simulink model "Pos_y_fza_P"  (R2021a)
settings: Solver=FixedStepAuto  StartTime=0.0  StopTime=Inf  FixedStep=0.01  RelTol=1e-3  EnableMultiTasking=on
libraries: arduinolib x7, cstblocks x1
settings Model: SILPILModeSetting=veronly  ExtModeTrigDuration=2  Creator=Simón  LastModifiedBy=Simón
settings OptimizationCC: EnhancedBackFolding=on  PassReuseOutputArgsAs=Individual arguments  ZeroExternalMemoryAtStartup=off  ZeroInternalMemoryAtStartup=off  MaxStackSize=64  OptimizeBlockOrder=speed  DifferentSizesBufferReuse=on  OptimizationCustomize=off  EfficientTunableParamExpr=on
settings DebuggingCC: ParameterTunabilityLossMsg=error
settings HardwareCC: ProdBitPerInt=16  ProdBitPerPointer=16  ProdBitPerSizeT=16  ProdBitPerPtrDiffT=16  ProdLargestAtomicFloat=None  ProdWordSize=8  ProdHWDeviceType=Atmel->AVR  UseEmbeddedCoderFeatures=off  UseSimulinkCoderFeatures=off
settings SFSimCC: MATLABDynamicMemAlloc=off
settings RTWCC: SystemTargetFile=ert.tlc  HardwareBoard=Arduino Uno  TemplateMakefile=ert_default_tmf  Toolchain=Arduino AVR  BuildConfiguration=Faster Runs
settings CodeAppCC: ForceParamTrailComments=on  IgnoreCustomStorageClasses=off  OperatorAnnotations=on  SimulinkDataObjDesc=on  SFDataObjDesc=on  InsertBlockDesc=on
settings ERTTargetCC: SupportContinuousTime=on  SupportNonInlinedSFcns=on  SupportVariableSizeSignals=on  ExtModeStaticAllocSize=250

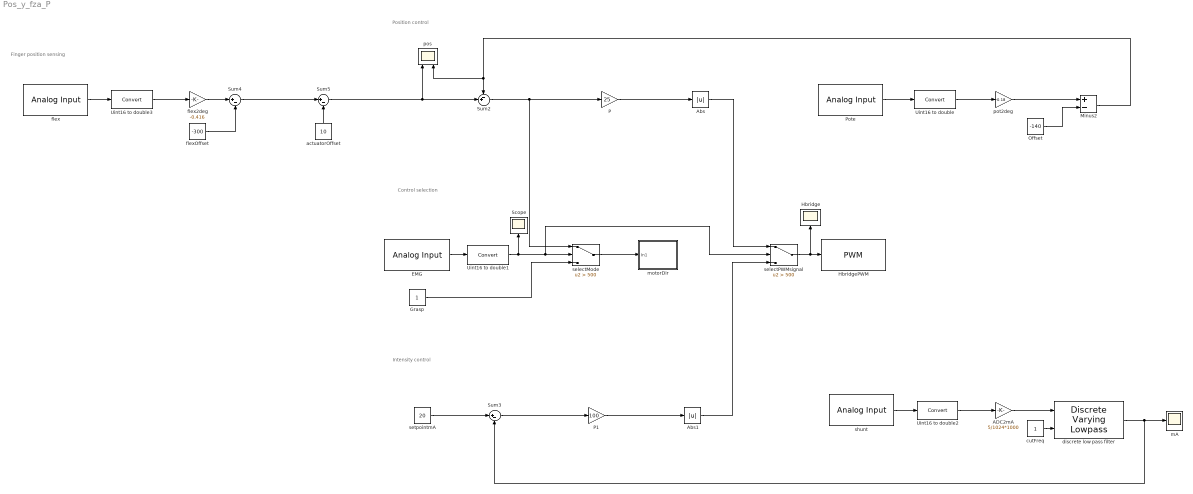
== system Pos_y_fza_P ==
  note: Finger position sensing
  note: Control selection
  note: Intensity control
  note: Position control
  ADC2mA : Gain  Gain=5/1024*1000
  Abs : Abs
  Abs1 : Abs
  EMG : arduinolib/Analog Input  pinNumber=5  ReadResultsOnly=off  ConversionTriggerSource=Software  ExternalTriggerType=uint32( 0 )  OutputDataType=uint16  EnableConversionCompleteNotify=off  EnableOuputStatus=off  SampleTime=-1  blockPlatform=arduino
  Grasp : Constant
  Hbridge : Scope
  HbridgePWM : arduinolib/PWM  pinNumber=10  frequencyType=Default  desiredFrequency=490.2  achievableFrequency=490.2
  Minus2 : Sum  Inputs=+-
  Offset : Constant  Value=-140
  P : Gain  Gain=25
  P1 : Gain  Gain=100
  Pote : arduinolib/Analog Input  pinNumber=0  ReadResultsOnly=off  ConversionTriggerSource=Software  ExternalTriggerType=uint32( 0 )  OutputDataType=uint16  EnableConversionCompleteNotify=off  EnableOuputStatus=off  SampleTime=-1  blockPlatform=arduino
  Scope : Scope
  Sum2 : Sum  Inputs=-+|
  Sum3 : Sum  Inputs=|+-
  Sum4 : Sum  Inputs=|+-
  Sum5 : Sum  Inputs=|+-
  Uint16 to double{,1..3} (4 alike) : DataTypeConversion
  actuatorOffset : Constant  Value=10
  cutFreq : Constant
  discrete low pass filter : cstblocks/Linear Parameter Varying/Discrete Varying Lowpass  N=1  w0=0  Ts=0.01
      settings: SourceProductBaseCode=CT
  flex : arduinolib/Analog Input  pinNumber=1  ReadResultsOnly=off  ConversionTriggerSource=Software  ExternalTriggerType=uint32( 0 )  OutputDataType=uint16  EnableConversionCompleteNotify=off  EnableOuputStatus=off  SampleTime=-1  blockPlatform=arduino
  flex2deg : Gain  Gain=-0.416
  flexOffset : Constant  Value=-300
  mA : Scope
  motorDir : Subsystem
  pos : Scope  NumInputPorts=2
  pot2deg : Gain  Gain=-0.18
  selectMode : Switch  Criteria=u2 > Threshold  Threshold=500
  selectPWMsignal : Switch  Criteria=u2 > Threshold  Threshold=500
  setpointmA : Constant  Value=20
  shunt : arduinolib/Analog Input  pinNumber=2  ReadResultsOnly=off  ConversionTriggerSource=Software  ExternalTriggerType=uint32( 0 )  OutputDataType=uint16  EnableConversionCompleteNotify=off  EnableOuputStatus=off  SampleTime=-1  blockPlatform=arduino
  wires:
  Pote/1 -> Uint16 to double/1
  Minus2/1 -> pos/2, Sum2/1
  Sum2/1 -> selectMode/1, P/1
  Abs/1 -> selectPWMsignal/1
  cutFreq/1 -> discrete low pass filter/2
  ADC2mA/1 -> discrete low pass filter/1
  discrete low pass filter/1 -> Sum3/2, mA/1
  shunt/1 -> Uint16 to double2/1
  Uint16 to double2/1 -> ADC2mA/1
  Uint16 to double/1 -> pot2deg/1
  pot2deg/1 -> Minus2/1
  selectMode/1 -> motorDir/1(In1)
  EMG/1 -> Uint16 to double1/1
  Uint16 to double1/1 -> Scope/1, selectPWMsignal/2, selectMode/2
  Grasp/1 -> selectMode/3
  selectPWMsignal/1 -> Hbridge/1, HbridgePWM/1
  Abs1/1 -> selectPWMsignal/3
  Sum3/1 -> P1/1
  setpointmA/1 -> Sum3/1
  flex2deg/1 -> Sum4/1
  flexOffset/1 -> Sum4/2
  flex/1 -> Uint16 to double3/1
  actuatorOffset/1 -> Sum5/2
  Offset/1 -> Minus2/2
  Uint16 to double3/1 -> flex2deg/1
  Sum4/1 -> Sum5/1
  Sum5/1 -> Sum2/2, pos/1
  P/1 -> Abs/1
  P1/1 -> Abs1/1

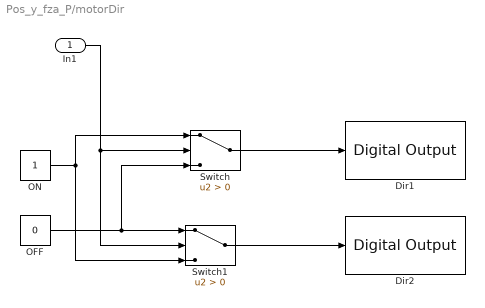
== system Pos_y_fza_P/motorDir ==
  In1 : Inport
  Dir1 : arduinolib/Digital Output  pinNumber=8  Direction=output  blockPlatform=arduino
  Dir2 : arduinolib/Digital Output  pinNumber=9  Direction=output  blockPlatform=arduino
  OFF : Constant  Value=0
  ON : Constant
  Switch : Switch  Criteria=u2 > Threshold
  Switch1 : Switch  Criteria=u2 > Threshold
  wires:
  In1/1 -> Switch1/2, Switch/2
  OFF/1 -> Switch/3, Switch1/1
  ON/1 -> Switch1/3, Switch/1
  Switch1/1 -> Dir2/1
  Switch/1 -> Dir1/1
